simulink model "execr2"  (R2016a)
settings: Solver=VariableStepAuto  StartTime=0.0  StopTime=10.0  RelTol=1e-3
values from neighbouring files (symbols this model uses):
  C1 = 170*10^-6    (= 0.00017)    [questao7.m]
  C2 = 170*10^-6    (= 0.00017)    [questao7.m]
  L = 2    [questao7.m]
  R1 = 25    [questao7.m]
  R2 = 25000    [questao7.m]
  R3 = 25000    [questao7.m]
settings Model: Creator=diona  LastModifiedBy=diona

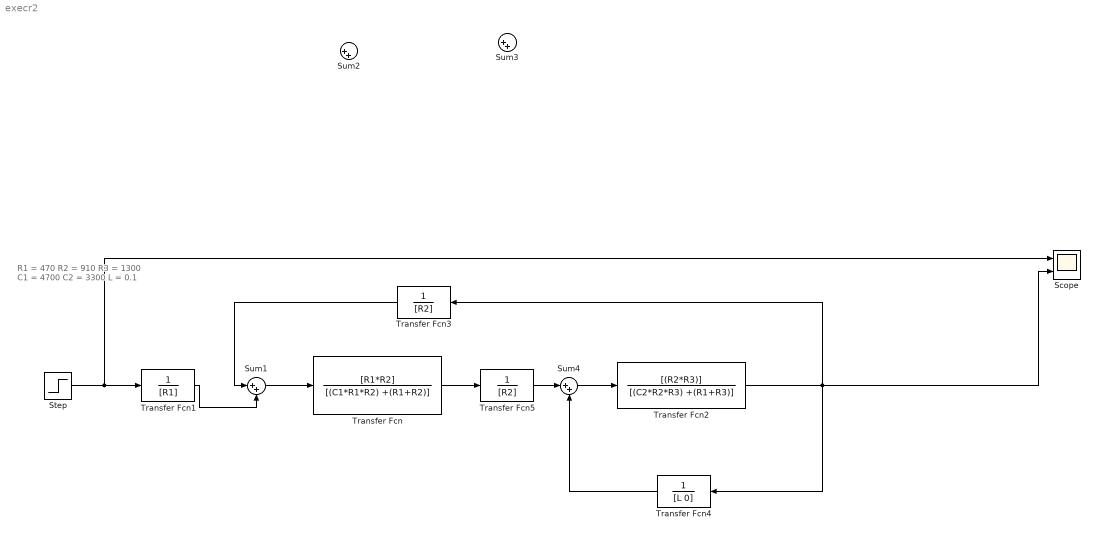
== system execr2 ==
  note: R1 = 470
      | R2 = 910
      | R3 = 1300
      |
      | C1 = 4700
      | C2 = 3300
      |
      | L = 0.1
  Scope : Scope  NumInputPorts=2
  Step : Step  SampleTime=0
  Sum{1..4} (4 alike) : Sum  Inputs=|++
  Transfer Fcn : TransferFcn  Numerator=[R1*R2]  Denominator=[(C1*R1*R2) +(R1+R2)]
  Transfer Fcn1 : TransferFcn  Denominator=[R1]
  Transfer Fcn2 : TransferFcn  Numerator=[(R2*R3)]  Denominator=[(C2*R2*R3) +(R1+R3)]
  Transfer Fcn3 : TransferFcn  Denominator=[R2]
  Transfer Fcn4 : TransferFcn  Denominator=[L 0]
  Transfer Fcn5 : TransferFcn  Denominator=[R2]
  wires:
  Sum4/1 -> Transfer Fcn2/1
  Transfer Fcn5/1 -> Sum4/1
  Transfer Fcn/1 -> Transfer Fcn5/1
  Sum1/1 -> Transfer Fcn/1
  Transfer Fcn1/1 -> Sum1/2
  Transfer Fcn4/1 -> Sum4/2
  Transfer Fcn3/1 -> Sum1/1
  Transfer Fcn2/1 -> Transfer Fcn3/1, Scope/2, Transfer Fcn4/1
  Step/1 -> Scope/1, Transfer Fcn1/1
